simulink model "transposed_direct_form_II"  (R2015a)
settings: Solver=ode45  StartTime=0.0  StopTime=10.0  RelTol=1e-3
undefined symbols (not defined in the file): sml_a1, sml_a2, sml_b0, sml_b1, sml_b2, sml_initial_states, sml_input_const, sml_prec_frac, sml_prec_int
libraries: simulink x1
settings Model: Creator=Lennon  LastModifiedBy=lennon
settings DebuggingCC: ParameterOverflowMsg=none  ParameterPrecisionLossMsg=none  ParameterTunabilityLossMsg=none

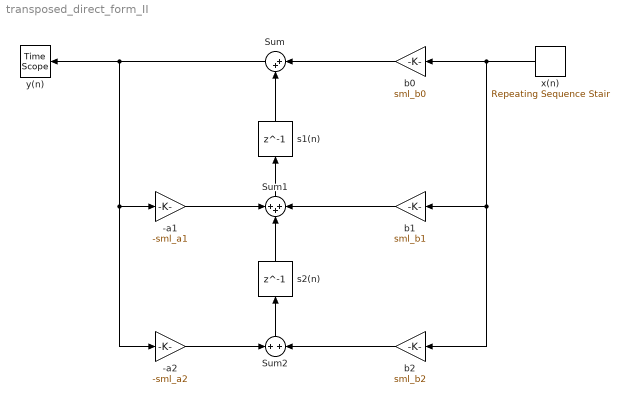
== system transposed_direct_form_II ==
  -a1 : Gain  Gain=-sml_a1  ParamDataTypeStr=fixdt(1,sml_prec_int+sml_prec_frac,sml_prec_frac)  OutDataTypeStr=fixdt(1,sml_prec_int+sml_prec_frac,sml_prec_frac)  RndMeth=Round
  -a2 : Gain  Gain=-sml_a2  ParamDataTypeStr=fixdt(1,sml_prec_int+sml_prec_frac,sml_prec_frac)  OutDataTypeStr=fixdt(1,sml_prec_int+sml_prec_frac,sml_prec_frac)  RndMeth=Round
  Sum : Sum  Inputs=|++  AccumDataTypeStr=fixdt(1,sml_prec_int+sml_prec_frac,sml_prec_frac)  OutDataTypeStr=fixdt(1,sml_prec_int+sml_prec_frac,sml_prec_frac)  RndMeth=Round
  Sum1 : Sum  Inputs=+++  AccumDataTypeStr=fixdt(1,sml_prec_int+sml_prec_frac,sml_prec_frac)  OutDataTypeStr=fixdt(1,sml_prec_int+sml_prec_frac,sml_prec_frac)  RndMeth=Round
  Sum2 : Sum  AccumDataTypeStr=fixdt(1,sml_prec_int+sml_prec_frac,sml_prec_frac)  OutDataTypeStr=fixdt(1,sml_prec_int+sml_prec_frac,sml_prec_frac)  RndMeth=Round
  b0 : Gain  Gain=sml_b0  ParamDataTypeStr=fixdt(1,sml_prec_int+sml_prec_frac,sml_prec_frac)  OutDataTypeStr=fixdt(1,sml_prec_int+sml_prec_frac,sml_prec_frac)  RndMeth=Round
  b1 : Gain  Gain=sml_b1  ParamDataTypeStr=fixdt(1,sml_prec_int+sml_prec_frac,sml_prec_frac)  OutDataTypeStr=fixdt(1,sml_prec_int+sml_prec_frac,sml_prec_frac)  RndMeth=Round
  b2 : Gain  Gain=sml_b2  ParamDataTypeStr=fixdt(1,sml_prec_int+sml_prec_frac,sml_prec_frac)  OutDataTypeStr=fixdt(1,sml_prec_int+sml_prec_frac,sml_prec_frac)  RndMeth=Round
  s1(n) : Delay  DelayLength=1  InitialCondition=norm(sml_initial_states)  SampleTime=1
  s2(n) : Delay  DelayLength=1  InitialCondition=norm(sml_initial_states)  SampleTime=1
  "x(n) " : simulink/Sources/Repeating Sequence Stair  OutValues=[sml_input_const sml_input_const sml_input_const sml_input_const sml_input_const sml_input_const sml_input_const sml_input_const sml_input_const sml_input_const]  tsamp=1  OutMin=[]  OutMax=[]  OutDataTypeStr=fixdt(1,sml_prec_int+sml_prec_frac,sml_prec_frac)  OutputDataTypeScalingMode=Specify via dialog  OutDataType=fixdt(1,sml_prec_int+sml_prec_frac,sml_prec_frac)  ConRadixGroup=Best Precision: Vector-wise  OutScaling=[]
  "y(n) " : TimeScope
  wires:
  s1(n)/1 -> Sum/2
  "x(n) "/1 -> b1/1, b2/1, b0/1
  b0/1 -> Sum/1
  Sum/1 -> "y(n) "/1, -a2/1, -a1/1
  s2(n)/1 -> Sum1/2
  -a1/1 -> Sum1/1
  b1/1 -> Sum1/3
  Sum1/1 -> s1(n)/1
  -a2/1 -> Sum2/1
  b2/1 -> Sum2/2
  Sum2/1 -> s2(n)/1
